simulink model "SystemModel"  (R2020a)
settings: Solver=VariableStepAuto  StartTime=0.0  StopTime=5  RelTol=1e-3
values from neighbouring files (symbols this model uses):
  D = 3.25    [MotorSpecMatFile.mat]    (also in SpecMotorMaxon.m = 0.093645)
  GR = 53    [MotorSpecMatFile.mat]    (also in SpecMotorMaxon.m)
  J = 8.2897999288e-05    [MotorSpecMatFile.mat]    (also in SpecMotorMaxon.m)
  kd = 40    [MotorSpecMatFile.mat]    (also in SpecMotorMaxon.m = 16)
  Ke = 0.0525    [MotorSpecMatFile.mat]    (also in SpecMotorMaxon.m)
  ke_I = 1.2    [MotorSpecMatFile.mat]    (also in SpecMotorMaxon.m = 1050.17921147)
  ki = 0.001    [MotorSpecMatFile.mat]    (also in SpecMotorMaxon.m = 1.389)
  ki_I = 1.2    [MotorSpecMatFile.mat]    (also in SpecMotorMaxon.m = 2100.35842294)
  Km = 0.0525    [MotorSpecMatFile.mat]
  kp = 65    [MotorSpecMatFile.mat]    (also in SpecMotorMaxon.m = 1.6)
  kp_I = 1    [MotorSpecMatFile.mat]    (also in SpecMotorMaxon.m = 2)
  Kt = 0.0525    [MotorSpecMatFile.mat]    (also in SpecMotorMaxon.m)
  L = 0.000279    [MotorSpecMatFile.mat]    (also in SpecMotorMaxon.m)
  maxI = 7.07106781187    [MotorSpecMatFile.mat]    (also in SpecMotorMaxon.m = 10/sqrt(2))
  maxV = 24    [MotorSpecMatFile.mat]    (also in SpecMotorMaxon.m)
  N = 12.3076923077    [MotorSpecMatFile.mat]    (also in SpecMotorMaxon.m = 170.858027658)
  R = 0.293    [MotorSpecMatFile.mat]    (also in SpecMotorMaxon.m)
  r = 5.79453537576e-05    [MotorSpecMatFile.mat]    (also in SpecMotorMaxon.m = Km*Io/(no*2*pi/60))
  RPM = 0    [MotorSpecMatFile.mat]    (also in SpecMotorMaxon.m)
undefined symbols (not defined in the file or in its folder): sigbuilder_block
libraries: simulink x1
settings Model: Creator=Dang Nguyen  LastModifiedBy=Dang Nguyen

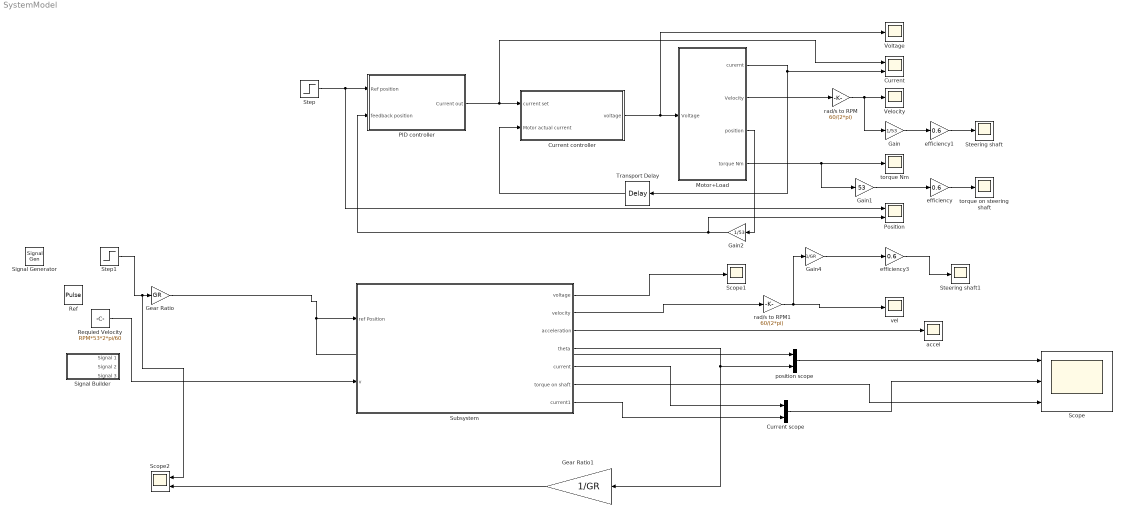
== system SystemModel ==
  Current : Scope  NumInputPorts=2
  Current controller : Subsystem
  Current scope : Mux  Inputs=2
  Gain : Gain  Gain=1/53
  Gain1 : Gain  Gain=53
  Gain2 : Gain  Gain=1/53
  Gain4 : Gain  Gain=1/GR
  Gear Ratio : Gain  Gain=GR
  Gear Ratio1 : Gain  Gain=1/GR
  Motor+Load : Subsystem
  PID controller : Subsystem
  Position : Scope  NumInputPorts=2
  Ref : DiscretePulseGenerator  PulseType=Time based  Amplitude=242/180*pi  Period=5  PulseWidth=50
  Requied Velocity : Constant  Value=RPM*53*2*pi/60
  Scope : Scope  NumInputPorts=3
  Scope1 : Scope
  Scope2 : Scope  NumInputPorts=2
  Signal Generator : SignalGenerator  Amplitude=120/180*pi  Frequency=0.2
  Signal Builder : Subsystem  Tag=STV Subsys  LoadFcn=sigbuilder_block('load');  StartFcn=sigbuilder_block('start');  StopFcn=sigbuilder_block('stop');  ClipboardFcn=sigbuilder_block('clipboard');  mask(Sigbuilder block){tuvar=[0:10]}
      mask help: Simulink:masks:SigbuilderBlock_MD
      mask init:
      | if ~strcmp(get_param(bdroot(gcbh),'SimulationStatus'),'stopped') tuvar = sigbuilder_block('maskInit'); end
      settings: CopyFcn=sigbuilder_block('copy');  DeleteFcn=sigbuilder_block('delete');  ModelCloseFcn=sigbuilder_block('modelClose');  PreSaveFcn=sigbuilder_block('preSave');  PauseFcn=sigbuilder_block('pause');  ContinueFcn=sigbuilder_block('continue');  NameChangeFcn=sigbuilder_block('namechange');  OpenFcn=sigbuilder_block('open',[437.6 199.2 550.4 400 ]);  CloseFcn=sigbuilder_block('close');
      mask Display: plot(0, 0, 100, 100,[2, 2, 32, 32, 2], [68, 8, 8, 68, 68],[32, 2], [38, 38], [32, 19, 2],[53, 60, 44], [32, 17, 17, 2],[16, 16, 31, 31]);txt = getActiveGroup(gcbh);text(2, 100, txt,'verticalAlignment', 'top');
  Steering shaft : Scope
  Steering shaft1 : Scope
  Step : Step  Time=0  After=242/180*pi  SampleTime=0
  Step1 : Step  SampleTime=0
  Subsystem : Subsystem
  Transport Delay : TransportDelay  DelayTime=0.06/1000
  Velocity : Scope
  Voltage : Scope
  accel : Scope
  efficiency : Gain  Gain=0.6
  efficiency1 : Gain  Gain=0.6
  efficiency3 : Gain  Gain=0.6
  position scope : Mux  Inputs=2
  rad/s to RPM : Gain  Gain=60/(2*pi)
  rad/s to RPM1 : Gain  Gain=60/(2*pi)
  torque Nm : Scope
  torque on steering shaft : Scope
  vel : Scope
  wires:
  Motor+Load/1(curernt) -> Current/2, Transport Delay/1
  Current controller/1(voltage) -> Motor+Load/1(Voltage), Voltage/1
  Transport Delay/1 -> Current controller/2(Motor actual current)
  Motor+Load/4(torque Nm) -> torque Nm/1, Gain1/1
  Motor+Load/2(Velocity) -> rad/s to RPM/1
  rad/s to RPM/1 -> Velocity/1, Gain/1
  PID controller/1(Current out) -> Current/1, Current controller/1(current set)
  efficiency/1 -> torque on steering shaft/1
  Gain1/1 -> efficiency/1
  efficiency1/1 -> Steering shaft/1
  Gain/1 -> efficiency1/1
  Motor+Load/3(position) -> Gain2/1
  Gain2/1 -> Position/2, PID controller/2(feedback position)
  rad/s to RPM1/1 -> vel/1, Gain4/1
  Gain4/1 -> efficiency3/1
  efficiency3/1 -> Steering shaft1/1
  Step/1 -> Position/1, PID controller/1(Ref position)
  Gear Ratio/1 -> position scope/1, Subsystem/1(ref Position)
  position scope/1 -> Scope/1
  Current scope/1 -> Scope/2
  Gear Ratio1/1 -> Scope2/2
  Subsystem/4(theta) -> Gear Ratio1/1, position scope/2
  Requied Velocity/1 -> Subsystem/2(v)
  Subsystem/1(voltage) -> Scope1/1
  Subsystem/2(velocity) -> rad/s to RPM1/1
  Subsystem/3(acceleration) -> accel/1
  Subsystem/5(current) -> Current scope/1
  Subsystem/6(torque on shaft) -> Scope/3
  Subsystem/7(current1) -> Current scope/2
  Step1/1 -> Scope2/1, Gear Ratio/1

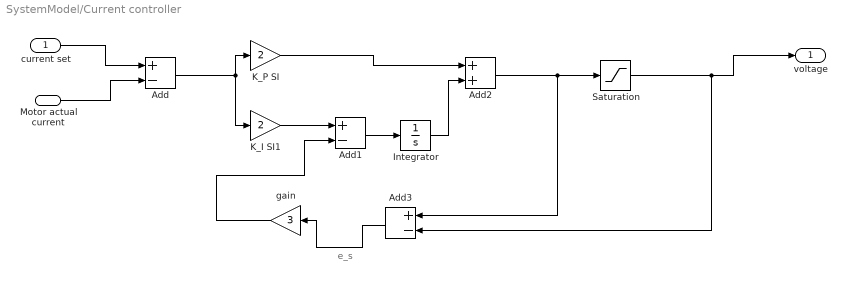
== system SystemModel/Current controller ==
  note: e_s
  current set : Inport
  Motor actual current : Inport  Port=2
  Add : Sum  Inputs=+-
  Add1 : Sum  Inputs=+-
  Add2 : Sum
  Add3 : Sum  Inputs=+-
  Integrator : Integrator
  K_I SI1 : Gain  Gain=2
  K_P SI : Gain  Gain=2
  Saturation : Saturate  UpperLimit=24  LowerLimit=-24
  gain : Gain  Gain=3
  voltage : Outport
  wires:
  Integrator/1 -> Add2/2
  Add1/1 -> Integrator/1
  K_I SI1/1 -> Add1/1
  Add/1 -> K_P SI/1, K_I SI1/1
  current set/1 -> Add/1
  K_P SI/1 -> Add2/1
  Add2/1 -> Saturation/1, Add3/1
  Motor actual current/1 -> Add/2
  Saturation/1 -> Add3/2, voltage/1
  Add3/1 -> gain/1
  gain/1 -> Add1/2

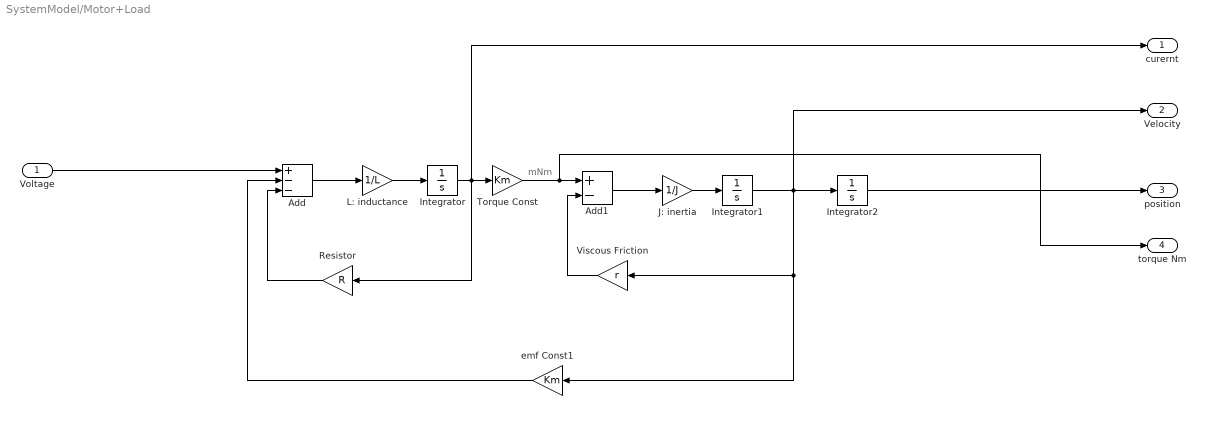
== system SystemModel/Motor+Load ==
  note: mNm
  Voltage : Inport
  Add : Sum  Inputs=+--
  Add1 : Sum  Inputs=+-
  Integrator : Integrator
  Integrator1 : Integrator
  Integrator2 : Integrator
  J: inertia : Gain  Gain=1/J
  L: inductance : Gain  Gain=1/L
  Resistor : Gain  Gain=R
  Torque Const : Gain  Gain=Km
  Viscous Friction : Gain  Gain=r
  emf Const1 : Gain  Gain=Km
  curernt : Outport
  Velocity : Outport  Port=2
  position : Outport  Port=3
  torque Nm : Outport  Port=4
  wires:
  Viscous Friction/1 -> Add1/2
  J: inertia/1 -> Integrator1/1
  L: inductance/1 -> Integrator/1
  Torque Const/1 -> Add1/1, torque Nm/1
  Add1/1 -> J: inertia/1
  Add/1 -> L: inductance/1
  Integrator/1 -> Torque Const/1, Resistor/1, curernt/1
  emf Const1/1 -> Add/2
  Resistor/1 -> Add/3
  Integrator2/1 -> position/1
  Integrator1/1 -> Velocity/1, Viscous Friction/1, emf Const1/1, Integrator2/1
  Voltage/1 -> Add/1

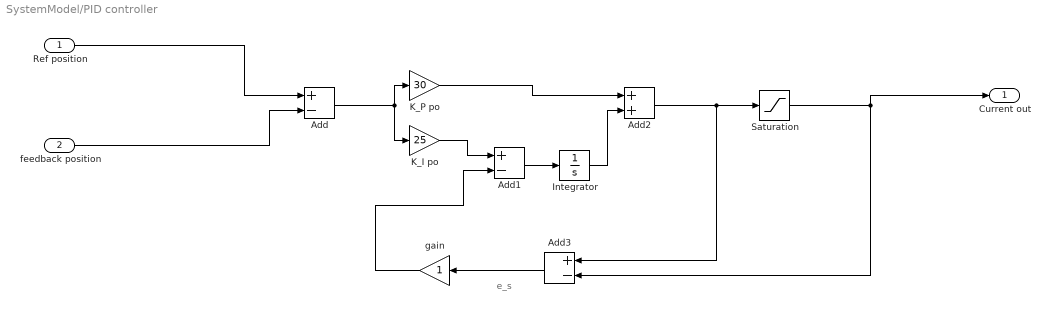
== system SystemModel/PID controller ==
  note: e_s
  Ref position : Inport
  feedback position : Inport  Port=2
  Add : Sum  Inputs=+-
  Add1 : Sum  Inputs=+-
  Add2 : Sum
  Add3 : Sum  Inputs=+-
  Integrator : Integrator
  K_I po : Gain  Gain=25
  K_P po : Gain  Gain=30
  Saturation : Saturate  UpperLimit=7.25  LowerLimit=-7.25
  gain : Gain
  Current out : Outport
  wires:
  gain/1 -> Add1/2
  Add3/1 -> gain/1
  Integrator/1 -> Add2/2
  Saturation/1 -> Current out/1, Add3/2
  Ref position/1 -> Add/1
  K_P po/1 -> Add2/1
  K_I po/1 -> Add1/1
  Add1/1 -> Integrator/1
  feedback position/1 -> Add/2
  Add/1 -> K_P po/1, K_I po/1
  Add2/1 -> Saturation/1, Add3/1

== system SystemModel/Signal Builder ==
  Demux : Demux  Tag=STV Demux  Outputs=3
      settings: DisplayOption=none
  FromWs : FromWorkspace  Tag=STV FromWs  VariableName=tuvar
      SigBuilderData=|
      | common.afterFinalStr = 'Extrapolate'
      | common.sampleTime = 0
      | dataSet.timeRange = [0 10]
      | dataSet.name = 'Group 1'
      | sbobj.Groups.Name = 'Group 1'
      | sbobj.Groups.Signals(1).Name = 'Signal 1'
      | sbobj.Groups.Signals(1).XData = [0 0.5 1 1.5 2.5 10]
      | sbobj.Groups.Signals(1).YData = [0 0.54 3.4 3.1 -1.57079632679 0]
      | sbobj.Groups.Signals(2).Name = 'Signal 2'
      | sbobj.Groups.Signals(2).XData = [0 5 5 10]
      | sbobj.Groups.Signals(2).YData = [0 0 1 1]
      | sbobj.Groups.Signals(3).Name = 'Signal 3'
      | sbobj.Groups.Signals(3).XData = [0 10]
      | sbobj.Groups.Signals(3).YData = [0 -0.02]
  Signal 1 : Outport  Tag=STV Outport
  Signal 2 : Outport  Tag=STV Outport  Port=2
  Signal 3 : Outport  Tag=STV Outport  Port=3
  wires:
  Demux/1 -> Signal 1/1
  FromWs/1 -> Demux/1
  Demux/2 -> Signal 2/1
  Demux/3 -> Signal 3/1

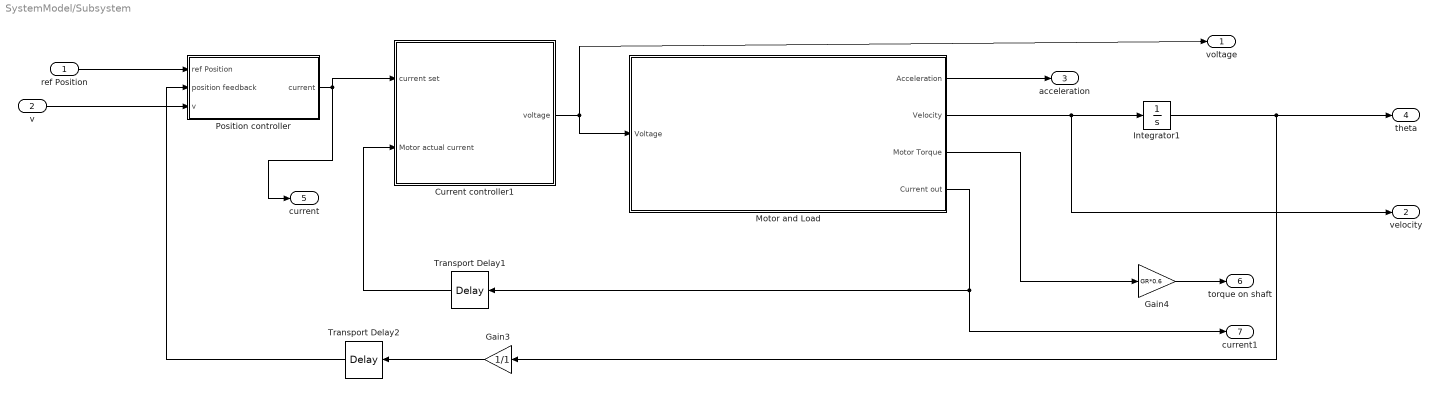
== system SystemModel/Subsystem ==
  ref Position : Inport
  v : Inport  Port=2
  Current controller1 : Subsystem
  Gain3 : Gain  Gain=1/1
  Gain4 : Gain  Gain=GR*0.6
  Integrator1 : Integrator
  Motor and Load : Subsystem
  Position controller : Subsystem
  Transport Delay1 : TransportDelay  DelayTime=0.06/1000
  Transport Delay2 : TransportDelay  DelayTime=0.4/1000
  voltage : Outport
  velocity : Outport  Port=2
  acceleration : Outport  Port=3
  theta : Outport  Port=4
  current : Outport  Port=5
  torque on shaft : Outport  Port=6
  current1 : Outport  Port=7
  wires:
  Transport Delay2/1 -> Position controller/2(position feedback)
  Gain3/1 -> Transport Delay2/1
  Transport Delay1/1 -> Current controller1/2(Motor actual current)
  Gain4/1 -> torque on shaft/1
  Integrator1/1 -> Gain3/1, theta/1
  Position controller/1(current) -> current/1, Current controller1/1(current set)
  v/1 -> Position controller/3(v)
  ref Position/1 -> Position controller/1(ref Position)
  Current controller1/1(voltage) -> Motor and Load/1(Voltage), voltage/1
  Motor and Load/4(Current out) -> current1/1, Transport Delay1/1
  Motor and Load/2(Velocity) -> Integrator1/1, velocity/1
  Motor and Load/1(Acceleration) -> acceleration/1
  Motor and Load/3(Motor Torque) -> Gain4/1

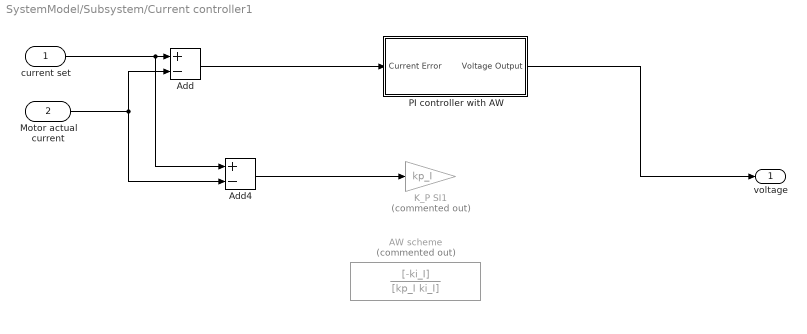
== system SystemModel/Subsystem/Current controller1 ==
  current set : Inport
  Motor actual current : Inport  Port=2
  AW scheme : TransferFcn  Commented=on  Numerator=[-ki_I]  Denominator=[kp_I ki_I]
  Add : Sum  Inputs=+-
  Add4 : Sum  Inputs=+-
  K_P SI1 : Gain  Commented=on  Gain=kp_I
  PI controller with AW : Subsystem
  voltage : Outport
  wires:
  current set/1 -> Add4/1, Add/1
  Motor actual current/1 -> Add4/2, Add/2
  Add4/1 -> K_P SI1/1
  Add/1 -> PI controller with AW/1(Current Error)
  PI controller with AW/1(Voltage Output) -> voltage/1

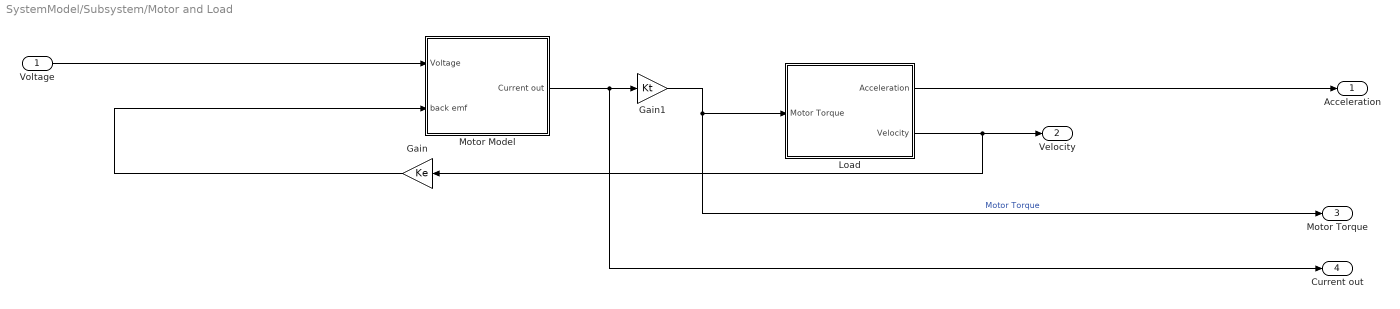
== system SystemModel/Subsystem/Motor and Load ==
  Voltage : Inport
  Gain : Gain  Gain=Ke
  Gain1 : Gain  Gain=Kt
  Load : Subsystem
  Motor Model : Subsystem
  Acceleration : Outport
  Velocity : Outport  Port=2
  Motor Torque : Outport  Port=3
  Current out : Outport  Port=4
  wires:
  Load/2(Velocity) -> Gain/1, Velocity/1
  Gain1/1 -> Motor Torque/1, Load/1(Motor Torque)  "Motor Torque"
  Load/1(Acceleration) -> Acceleration/1
  Voltage/1 -> Motor Model/1(Voltage)
  Gain/1 -> Motor Model/2(back emf)
  Motor Model/1(Current out) -> Current out/1, Gain1/1

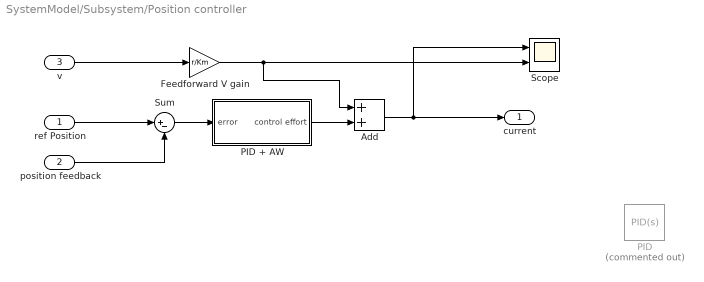
== system SystemModel/Subsystem/Position controller ==
  ref Position : Inport
  position feedback : Inport  Port=2
  v : Inport  Port=3
  Add : Sum
  Feedforward V gain : Gain  Gain=r/Km
  PID : simulink/Continuous/PID Controller  Commented=on  Controller=PID  Form=Parallel  TimeDomain=Continuous-time  UseExternalTs=off  SampleTime=-1  IntegratorMethod=Forward Euler  FilterMethod=Forward Euler  ControllerParametersSource=internal  P=kp  I=ki  D=D  UseFilter=on  N=N  TunerSelectOption=Transfer Function Based (PID Tuner App)  InitialConditionSource=internal  InitialConditionForIntegrator=0  InitialConditionForFilter=0  DifferentiatorICPrevScaledInput=0  ExternalReset=none  TrackingMode=off  Kt=1  LimitOutput=off  UpperSaturationLimit=inf  LowerSaturationLimit=-inf  LinearizeAsGain=on  AntiWindupMode=none  Kb=1  POutMin=[]  POutMax=[]  IOutMin=[]  IOutMax=[]  DOutMin=[]  DOutMax=[]  NOutMin=[]  NOutMax=[]  SumOutMin=[]  SumOutMax=[]  SaturationOutMin=[]  SaturationOutMax=[]  PParamMin=[]  PParamMax=[]  IParamMin=[]  IParamMax=[]  DParamMin=[]  DParamMax=[]  NParamMin=[]  NParamMax=[]  KbParamMin=[]  KbParamMax=[]  KtParamMin=[]  KtParamMax=[]  KbOutMin=[]  KbOutMax=[]  KtOutMin=[]  KtOutMax=[]  IntegratorOutMin=[]  IntegratorOutMax=[]  FilterOutMin=[]  FilterOutMax=[]  SumI1OutMin=[]  SumI1OutMax=[]  SumI2OutMin=[]  SumI2OutMax=[]  SumI3OutMin=[]  SumI3OutMax=[]  SumI4OutMin=[]  SumI4OutMax=[]  SumDOutMin=[]  SumDOutMax=[]  DifferentiatorOutMin=[]  DifferentiatorOutMax=[]  FilterDiffOutCoefMin=[]  FilterDiffOutCoefMax=[]  ReciprocalOutMin=[]  ReciprocalOutMax=[]  SumDenOutMin=[]  SumDenOutMax=[]  SumNumOutMin=[]  SumNumOutMax=[]  DivideOutMin=[]  DivideOutMax=[]  UdiffTsProdOutMin=[]  UdiffTsProdOutMax=[]  NTsProdOutMin=[]  NTsProdOutMax=[]  UintegralTsProdOutMin=[]  UintegralTsProdOutMax=[]  UngainTsProdOutMin=[]  UngainTsProdOutMax=[]  IntegratorContinuousStateAttributes=''  IntegratorStateMustResolveToSignalObject=off  IntegratorRTWStateStorageClass=Auto  FilterContinuousStateAttributes=''  FilterStateMustResolveToSignalObject=off  FilterRTWStateStorageClass=Auto  ParallelPVariant=InternalParameters  IdealPVariant=Disabled  IVariant=InternalParameters  DVariant=InternalParameters  IntegratorVariant=Continuous  SatVariant=Disabled  AWVariant=Passthrough  PCopyVariant=Disabled  TRVariant=Disabled  FdbkBlocksVariant=Forward  IdealPFdbkVariant=Disabled  SatFdbkVariant=Disabled  DerivativeFilterVariant=ContFilter  NVariant=InternalParameters  NCopyVariant=Disabled  FilterICVariant=InternalICsFilter  IntegratorICVariant=InternalICs  ExternalResetVariant=Disabled  TRSumVariant=Passthrough  SumFdbkVariant=Disabled  SumVariant=Sum_PID  TsampFilterVariant=InternalTs  TsampNgainVariant=Passthrough  TsampIntegralVariant=Passthrough
  PID + AW : Subsystem
  Scope : Scope  NumInputPorts=2
  Sum : Sum  Inputs=|+-
  current : Outport
  wires:
  position feedback/1 -> Sum/2
  ref Position/1 -> Sum/1
  Sum/1 -> PID + AW/1(error)
  Add/1 -> current/1, Scope/1
  Feedforward V gain/1 -> Scope/2, Add/1
  PID + AW/1(control effort) -> Add/2
  v/1 -> Feedforward V gain/1

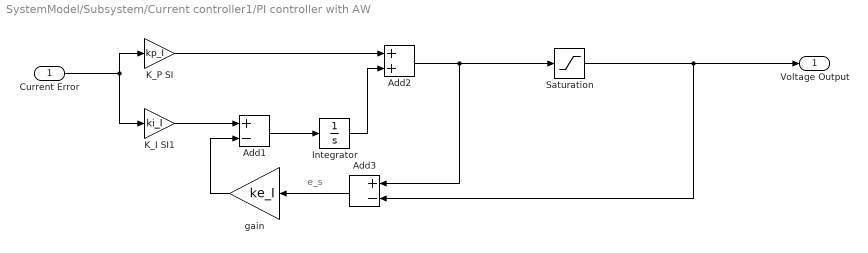
== system SystemModel/Subsystem/Current controller1/PI controller with AW ==
  note: e_s
  Current Error : Inport
  Add1 : Sum  Inputs=+-
  Add2 : Sum
  Add3 : Sum  Inputs=+-
  Integrator : Integrator
  K_I SI1 : Gain  Gain=ki_I
  K_P SI : Gain  Gain=kp_I
  Saturation : Saturate  UpperLimit=maxV  LowerLimit=-maxV
  gain : Gain  Gain=ke_I
  Voltage Output : Outport
  wires:
  Current Error/1 -> K_P SI/1, K_I SI1/1
  Add1/1 -> Integrator/1
  Add2/1 -> Saturation/1, Add3/1
  Integrator/1 -> Add2/2
  Add3/1 -> gain/1
  K_I SI1/1 -> Add1/1
  gain/1 -> Add1/2
  Saturation/1 -> Voltage Output/1, Add3/2
  K_P SI/1 -> Add2/1

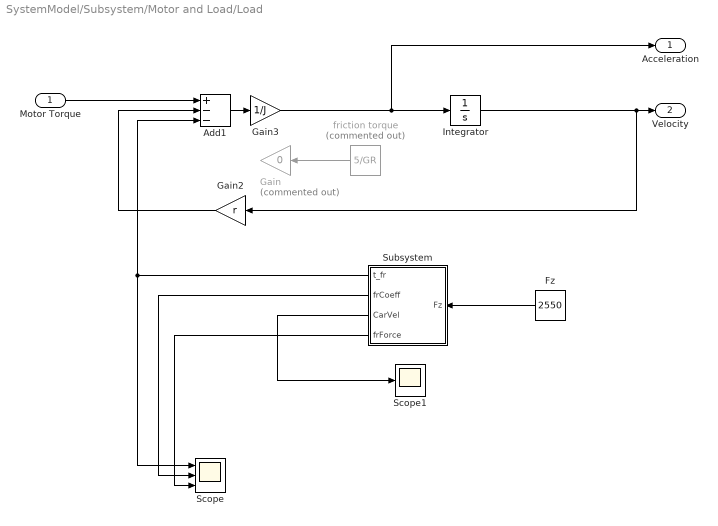
== system SystemModel/Subsystem/Motor and Load/Load ==
  Motor Torque : Inport
  Add1 : Sum  Inputs=+--
  Fz : Constant  Value=2550
  Gain : Gain  Commented=on  Gain=0
  Gain2 : Gain  Gain=r
  Gain3 : Gain  Gain=1/J
  Integrator : Integrator
  Scope : Scope  NumInputPorts=3
  Scope1 : Scope
  Subsystem : Subsystem
  friction torque : Constant  Commented=on  Value=5/GR
  Acceleration : Outport
  Velocity : Outport  Port=2
  wires:
  Add1/1 -> Gain3/1
  Integrator/1 -> Gain2/1, Velocity/1
  Gain2/1 -> Add1/2
  Gain3/1 -> Acceleration/1, Integrator/1
  Motor Torque/1 -> Add1/1
  friction torque/1 -> Gain/1
  Subsystem/1(t_fr) -> Scope/1, Add1/3
  Fz/1 -> Subsystem/1(Fz)
  Subsystem/2(frCoeff) -> Scope/2
  Subsystem/3(CarVel) -> Scope1/1
  Subsystem/4(frForce) -> Scope/3

== system SystemModel/Subsystem/Motor and Load/Motor Model ==
  Voltage : Inport
  back emf : Inport  Port=2
  Add : Sum  Inputs=+-
  Saturation : Saturate  UpperLimit=10/sqrt(2)  LowerLimit=-10/sqrt(2)
  Transfer Fcn : TransferFcn  Denominator=[L R]
  Current out : Outport
  wires:
  Add/1 -> Transfer Fcn/1
  Voltage/1 -> Add/1
  back emf/1 -> Add/2
  Transfer Fcn/1 -> Saturation/1
  Saturation/1 -> Current out/1

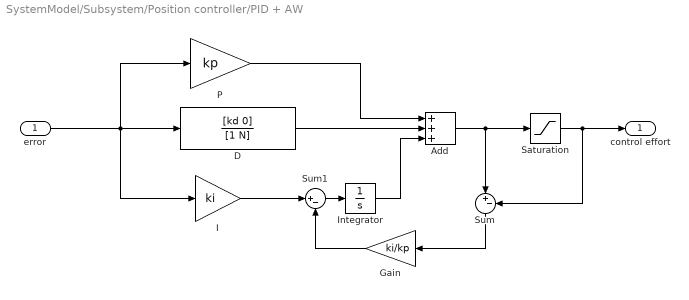
== system SystemModel/Subsystem/Position controller/PID + AW ==
  error : Inport
  Add : Sum  Inputs=+++
  D : TransferFcn  Numerator=[kd 0]  Denominator=[1 N]
  Gain : Gain  Gain=ki/kp
  I : Gain  Gain=ki
  Integrator : Integrator
  P : Gain  Gain=kp
  Saturation : Saturate  UpperLimit=maxI  LowerLimit=-maxI
  Sum : Sum  Inputs=|+-
  Sum1 : Sum  Inputs=|+-
  control effort : Outport
  wires:
  error/1 -> I/1, D/1, P/1
  Add/1 -> Saturation/1, Sum/1
  Saturation/1 -> Sum/2, control effort/1
  I/1 -> Sum1/1
  Gain/1 -> Sum1/2
  Sum/1 -> Gain/1
  Sum1/1 -> Integrator/1
  Integrator/1 -> Add/3
  D/1 -> Add/2
  P/1 -> Add/1

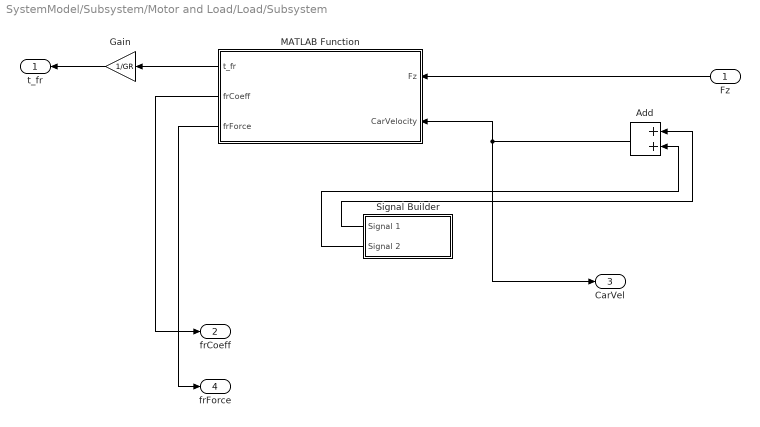
== system SystemModel/Subsystem/Motor and Load/Load/Subsystem ==
  Fz : Inport
  Add : Sum
  Gain : Gain  Gain=1/GR
  MATLAB Function : MATLAB Function  TreatAsAtomicUnit=on
  Signal Builder : Subsystem  Tag=STV Subsys  LoadFcn=sigbuilder_block('load');  StartFcn=sigbuilder_block('start');  StopFcn=sigbuilder_block('stop');  ClipboardFcn=sigbuilder_block('clipboard');  mask(Sigbuilder block){tuvar=[0:10]}
      mask help: Simulink:masks:SigbuilderBlock_MD
      mask init:
      | if ~strcmp(get_param(bdroot(gcbh),'SimulationStatus'),'stopped') tuvar = sigbuilder_block('maskInit'); end
      settings: CopyFcn=sigbuilder_block('copy');  DeleteFcn=sigbuilder_block('delete');  ModelCloseFcn=sigbuilder_block('modelClose');  PreSaveFcn=sigbuilder_block('preSave');  PauseFcn=sigbuilder_block('pause');  ContinueFcn=sigbuilder_block('continue');  NameChangeFcn=sigbuilder_block('namechange');  OpenFcn=sigbuilder_block('open',[437.6 199.2 550.4 400 ]);  CloseFcn=sigbuilder_block('close');
      mask Display: plot(0, 0, 100, 100,[2, 2, 32, 32, 2], [68, 8, 8, 68, 68],[32, 2], [38, 38], [32, 19, 2],[53, 60, 44], [32, 17, 17, 2],[16, 16, 31, 31]);txt = getActiveGroup(gcbh);text(2, 100, txt,'verticalAlignment', 'top');
  t_fr : Outport
  frCoeff : Outport  Port=2
  CarVel : Outport  Port=3
  frForce : Outport  Port=4
  wires:
  Signal Builder/2(Signal 2) -> Add/2
  Fz/1 -> MATLAB Function/1(Fz)
  Signal Builder/1(Signal 1) -> Add/1
  Add/1 -> CarVel/1, MATLAB Function/2(CarVelocity)
  MATLAB Function/2(frCoeff) -> frCoeff/1
  MATLAB Function/3(frForce) -> frForce/1
  Gain/1 -> t_fr/1
  MATLAB Function/1(t_fr) -> Gain/1

== system SystemModel/Subsystem/Motor and Load/Load/Subsystem/Signal Builder ==
  Demux : Demux  Tag=STV Demux  Outputs=2
      settings: DisplayOption=none
  FromWs : FromWorkspace  Tag=STV FromWs  VariableName=tuvar
      SigBuilderData=|
      | common.afterFinalStr = 'Extrapolate'
      | common.sampleTime = 0
      | dataSet.timeRange = [0 10]
      | dataSet.name = 'Group 1'
      | sbobj.Groups.Name = 'Group 1'
      | sbobj.Groups.Signals(1).Name = 'Signal 1'
      | sbobj.Groups.Signals(1).XData = [0 0.5 0.5 1 1.5 2.5 10]
      | sbobj.Groups.Signals(1).YData = [0.05 6.9 7.1 7.05 7.05 7.1 7.2]
      | sbobj.Groups.Signals(2).Name = 'Signal 2'
      | sbobj.Groups.Signals(2).XData = [0 5 5 10]
      | sbobj.Groups.Signals(2).YData = [0 0 1 1]
  Signal 1 : Outport  Tag=STV Outport
  Signal 2 : Outport  Tag=STV Outport  Port=2
  wires:
  Demux/1 -> Signal 1/1
  FromWs/1 -> Demux/1
  Demux/2 -> Signal 2/1

== matlab function SystemModel/Subsystem/Motor and Load/Load/Subsystem/MATLAB Function ==
  data: Fz input; t_fr output; CarVelocity input; frCoeff output; frForce output
function [t_fr,frCoeff, frForce] = frictionTorqueOnShaft(Fz,CarVelocity)

% CarVelocity: km/h
    
mechTrail = 9.599;          % (mm)
b = 82.2;                      % Longitudinal tie rod offset (mm)
pinionRadi = 0.039/2;

frCoeff = 0.451 * exp(-0.4603*CarVelocity) + 0.2376;  % friction coefficient from Study on Low-Speed Steering Resistance Torque of Vehicles Considering Friction between Tire and Pavement - eq (1) page 6
frForce = frCoeff*Fz;

t_fr = pinionRadi *  2*frForce*mechTrail/b;  % Ref: Design and implementation of an Electric Power Steering system for a Formula Student Driverless vehicle - pg31
